simulink model "hems_model"  (R2024b)
settings: Solver=ode3  StartTime=0.0  StopTime=86400  FixedStep=900  RelTol=1e-3
values from neighbouring files (symbols this model uses):
  A_win = 15    [hems_init.m]
  bat_cap = 10000    [hems_init.m]
  bat_eff_1way = sqrt(bat_eff)    [hems_init.m]
  bat_soc0 = 5000    [hems_init.m]
  C_bldg = 8000 * 3600    (= 28800000)    [hems_init.m]
  C_tank = V_tank*rho_w*c_w    (= 1255800)    [hems_init.m]
  dr_power = 2500    [hems_init.m]
  g_val = 0.55    [hems_init.m]
  H_T = 128    [hems_init.m]
  Q_int = 600    [hems_init.m]
  T_in0 = 20    [hems_init.m]
  T_tank0 = 55    [hems_init.m]
  UA_tank = 2.5    [hems_init.m]
  wm_power = 1500    [hems_init.m]
libraries: simulink x2
settings Model: Creator=orakanti1997  LastModifiedBy=orakanti1997

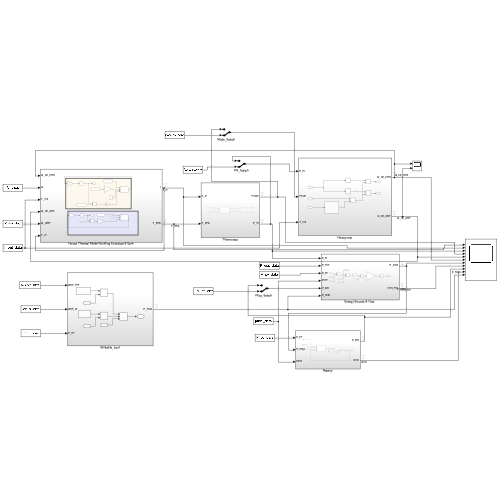
[thumbnail: Simulink's stored preview of the top-level diagram]
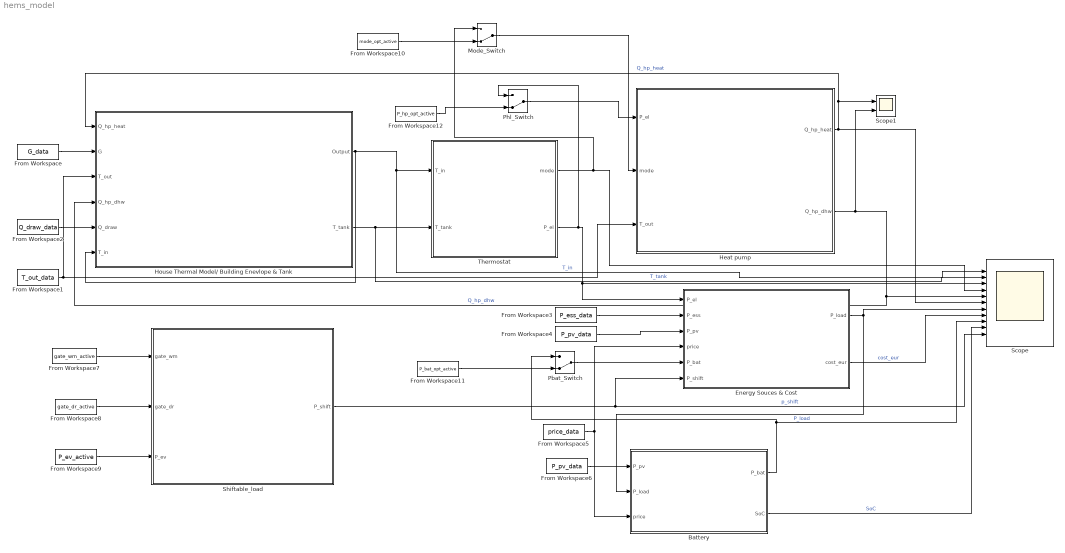
== system hems_model ==
  Battery : Subsystem
  "Energy Souces & Cost " : Subsystem
  From Workspace : FromWorkspace  VariableName=G_data  SampleTime=900
  From Workspace1 : FromWorkspace  VariableName=T_out_data  SampleTime=900
  From Workspace10 : FromWorkspace  VariableName=mode_opt_active
  From Workspace11 : FromWorkspace  VariableName=P_bat_opt_active
  From Workspace12 : FromWorkspace  VariableName=P_hp_opt_active
  From Workspace2 : FromWorkspace  VariableName=Q_draw_data  SampleTime=900
  From Workspace3 : FromWorkspace  VariableName=P_ess_data
  From Workspace4 : FromWorkspace  VariableName=P_pv_data
  From Workspace5 : FromWorkspace  VariableName=price_data
  From Workspace6 : FromWorkspace  VariableName=P_pv_data
  From Workspace7 : FromWorkspace  VariableName=gate_wm_active
  From Workspace8 : FromWorkspace  VariableName=gate_dr_active
  From Workspace9 : FromWorkspace  VariableName=P_ev_active
  Heat pump : Subsystem
  House Thermal Model/ Building Enevlope & Tank : Subsystem
  Mode_Switch : ManualSwitch  CurrentSetting=0
  Pbat_Switch : ManualSwitch  CurrentSetting=0
  Phl_Switch : ManualSwitch  CurrentSetting=0
  Scope : Scope  NumInputPorts=11
  Scope1 : Scope  NumInputPorts=2
  Shiftable_load : Subsystem
  Thermostat : Subsystem
  wires:
  Battery/1(P_bat) -> Pbat_Switch/1, Scope/9
  "Energy Souces & Cost "/2(cost_eur) -> Scope/8  "cost_eur"
  Heat pump/2(Q_hp_dhw) -> House Thermal Model/ Building Enevlope & Tank/4(Q_hp_dhw), Scope/5, Scope1/2  "Q_hp_dhw"
  Shiftable_load/1(P_shift) -> "Energy Souces & Cost "/6(P_shift), Scope/11  "p_shift"
  From Workspace5/1 -> "Energy Souces & Cost "/4(price), Battery/3(price)
  From Workspace4/1 -> "Energy Souces & Cost "/3(P_pv)
  "Energy Souces & Cost "/1(P_load) -> Battery/2(P_load), Scope/7  "P_load"
  Heat pump/1(Q_hp_heat) -> Scope1/1, House Thermal Model/ Building Enevlope & Tank/1(Q_hp_heat), Scope/6  "Q_hp_heat"
  From Workspace/1 -> House Thermal Model/ Building Enevlope & Tank/2(G)
  From Workspace3/1 -> "Energy Souces & Cost "/2(P_ess)
  From Workspace6/1 -> Battery/1(P_pv)
  Thermostat/1(mode) -> Mode_Switch/1, Scope/4
  From Workspace9/1 -> Shiftable_load/3(P_ev)
  From Workspace7/1 -> Shiftable_load/1(gate_wm)
  House Thermal Model/ Building Enevlope & Tank/2(T_tank) -> Thermostat/2(T_tank), Scope/2  "T_tank"
  From Workspace8/1 -> Shiftable_load/2(gate_dr)
  House Thermal Model/ Building Enevlope & Tank/1(Output) -> Thermostat/1(T_in), Scope/1, House Thermal Model/ Building Enevlope & Tank/6(T_in)  "T_in"
  Thermostat/2(P_el) -> Phl_Switch/1, Scope/3, "Energy Souces & Cost "/1(P_el)
  From Workspace1/1 -> Heat pump/3(T_out), House Thermal Model/ Building Enevlope & Tank/3(T_out)
  Battery/2(SoC) -> Scope/10  "SoC"
  From Workspace2/1 -> House Thermal Model/ Building Enevlope & Tank/5(Q_draw)
  Mode_Switch/1 -> Heat pump/2(mode)
  From Workspace10/1 -> Mode_Switch/2
  Pbat_Switch/1 -> "Energy Souces & Cost "/5(P_bat)
  From Workspace11/1 -> Pbat_Switch/2
  Phl_Switch/1 -> Heat pump/1(P_el)
  From Workspace12/1 -> Phl_Switch/2

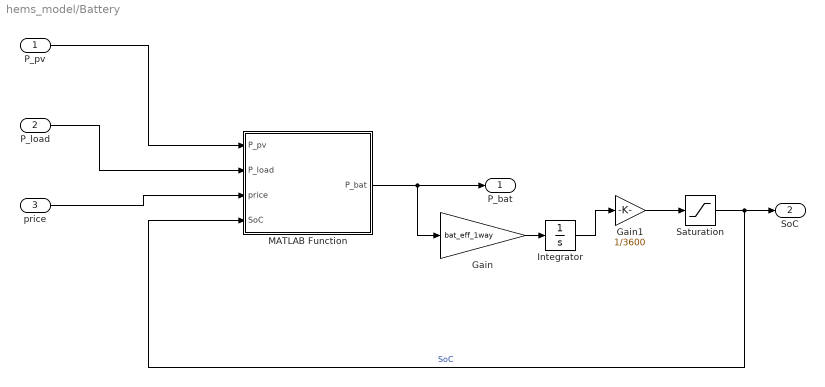
== system hems_model/Battery ==
  P_pv : Inport
  P_load : Inport  Port=2
  price : Inport  Port=3
  Gain : Gain  Gain=bat_eff_1way
  Gain1 : Gain  Gain=1/3600
  Integrator : Integrator  InitialCondition=bat_soc0
  MATLAB Function : MATLAB Function  TreatAsAtomicUnit=on
  Saturation : Saturate  UpperLimit=0.95*bat_cap  LowerLimit=0.10*bat_cap
  P_bat : Outport
  SoC : Outport  Port=2
  wires:
  P_pv/1 -> MATLAB Function/1(P_pv)
  P_load/1 -> MATLAB Function/2(P_load)
  price/1 -> MATLAB Function/3(price)
  Saturation/1 -> MATLAB Function/4(SoC), SoC/1  "SoC"
  MATLAB Function/1(P_bat) -> Gain/1, P_bat/1
  Integrator/1 -> Gain1/1
  Gain1/1 -> Saturation/1
  Gain/1 -> Integrator/1

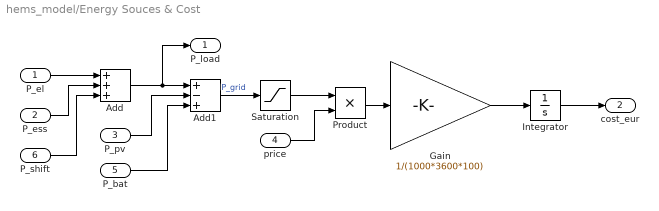
== system hems_model/Energy Souces & Cost  ==
  P_el : Inport
  P_ess : Inport  Port=2
  P_pv : Inport  Port=3
  price : Inport  Port=4
  P_bat : Inport  Port=5
  P_shift : Inport  Port=6
  Add : Sum  Inputs=+++
  Add1 : Sum  Inputs=+-+
  Gain : Gain  Gain=1/(1000*3600*100)
  Integrator : Integrator
  Product : Product
  Saturation : Saturate  UpperLimit=inf  LowerLimit=0
  P_load : Outport
  cost_eur : Outport  Port=2
  wires:
  Product/1 -> Gain/1
  price/1 -> Product/2
  Saturation/1 -> Product/1
  Integrator/1 -> cost_eur/1
  P_pv/1 -> Add1/2
  Gain/1 -> Integrator/1
  P_bat/1 -> Add1/3
  Add/1 -> P_load/1, Add1/1
  P_shift/1 -> Add/3
  P_ess/1 -> Add/2
  Add1/1 -> Saturation/1  "P_grid"
  P_el/1 -> Add/1

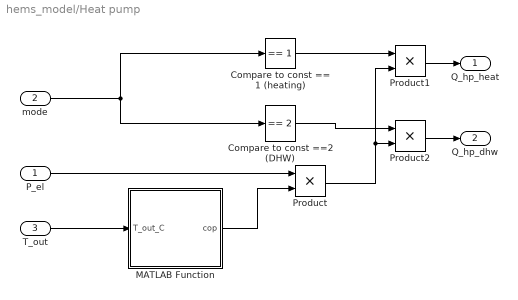
== system hems_model/Heat pump ==
  P_el : Inport
  mode : Inport  Port=2
  T_out : Inport  Port=3
  Compare to const == 1 (heating) : simulink/Logic and Bit Operations/Compare To Constant  relop===  const=1  OutDataTypeStr=uint8
  "Compare to const ==2 (DHW) " : simulink/Logic and Bit Operations/Compare To Constant  relop===  const=2  OutDataTypeStr=uint8
  MATLAB Function : MATLAB Function  TreatAsAtomicUnit=on
  Product : Product
  Product1 : Product
  Product2 : Product
  Q_hp_heat : Outport
  Q_hp_dhw : Outport  Port=2
  wires:
  Product1/1 -> Q_hp_heat/1
  Product/1 -> Product1/2, Product2/2
  Product2/1 -> Q_hp_dhw/1
  MATLAB Function/1(cop) -> Product/2
  Compare to const == 1 (heating)/1 -> Product1/1
  "Compare to const ==2 (DHW) "/1 -> Product2/1
  P_el/1 -> Product/1
  mode/1 -> Compare to const == 1 (heating)/1, "Compare to const ==2 (DHW) "/1
  T_out/1 -> MATLAB Function/1(T_out_C)

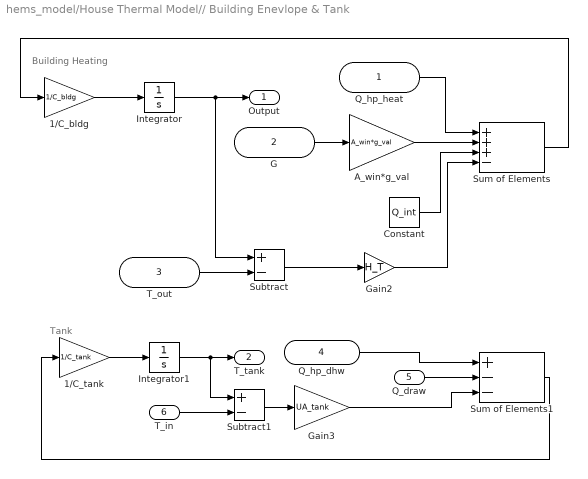
== system hems_model/House Thermal Model// Building Enevlope & Tank ==
  note: Building Heating
  note: Tank
  Q_hp_heat : Inport
  G : Inport  Port=2
  T_out : Inport  Port=3
  Q_hp_dhw : Inport  Port=4
  Q_draw : Inport  Port=5
  T_in : Inport  Port=6
  1/C_bldg : Gain  Gain=1/C_bldg
  1/C_tank : Gain  Gain=1/C_tank
  A_win*g_val : Gain  Gain=A_win*g_val
  Constant : Constant  Value=Q_int
  Gain2 : Gain  Gain=H_T
  Gain3 : Gain  Gain=UA_tank
  Integrator : Integrator  InitialCondition=T_in0
  Integrator1 : Integrator  InitialCondition=T_tank0
  Subtract : Sum  Inputs=+-
  Subtract1 : Sum  Inputs=+-
  Sum of Elements : Sum  Inputs=+++-
  Sum of Elements1 : Sum  Inputs=+--
  Output : Outport
  T_tank : Outport  Port=2
  wires:
  Gain2/1 -> Sum of Elements/4
  A_win*g_val/1 -> Sum of Elements/2
  Q_hp_heat/1 -> Sum of Elements/1
  Subtract/1 -> Gain2/1
  G/1 -> A_win*g_val/1
  Integrator/1 -> Subtract/1, Output/1
  Constant/1 -> Sum of Elements/3
  Sum of Elements1/1 -> 1/C_tank/1
  Q_draw/1 -> Sum of Elements1/2
  Gain3/1 -> Sum of Elements1/3
  Q_hp_dhw/1 -> Sum of Elements1/1
  Sum of Elements/1 -> 1/C_bldg/1
  Subtract1/1 -> Gain3/1
  1/C_bldg/1 -> Integrator/1
  Integrator1/1 -> Subtract1/1, T_tank/1
  T_in/1 -> Subtract1/2
  T_out/1 -> Subtract/2
  1/C_tank/1 -> Integrator1/1

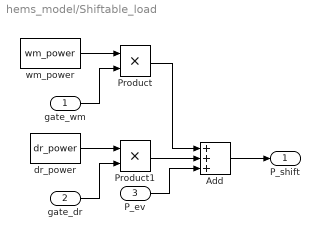
== system hems_model/Shiftable_load ==
  gate_wm : Inport
  gate_dr : Inport  Port=2
  P_ev : Inport  Port=3
  Add : Sum  Inputs=+++
  Product : Product
  Product1 : Product
  dr_power : Constant  Value=dr_power
  wm_power : Constant  Value=wm_power
  P_shift : Outport
  wires:
  P_ev/1 -> Add/3
  Product1/1 -> Add/2
  gate_dr/1 -> Product1/2
  dr_power/1 -> Product1/1
  Add/1 -> P_shift/1
  Product/1 -> Add/1
  gate_wm/1 -> Product/2
  wm_power/1 -> Product/1

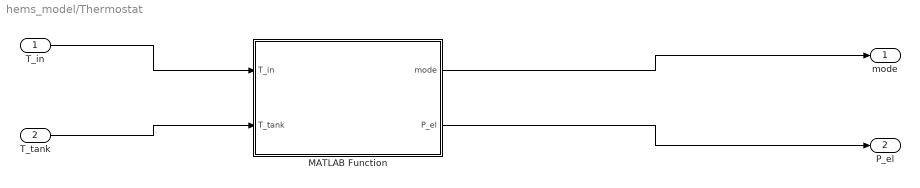
== system hems_model/Thermostat ==
  T_in : Inport
  T_tank : Inport  Port=2
  MATLAB Function : MATLAB Function  TreatAsAtomicUnit=on
  mode : Outport
  P_el : Outport  Port=2
  wires:
  T_in/1 -> MATLAB Function/1(T_in)
  T_tank/1 -> MATLAB Function/2(T_tank)
  MATLAB Function/1(mode) -> mode/1
  MATLAB Function/2(P_el) -> P_el/1

== matlab function hems_model/Thermostat/MATLAB Function ==
  data: T_in input; mode output; T_tank input; P_el output
function [mode, P_el] = thermostat(T_in, T_tank)
    % Rule-based thermostat controller
    % Priority: hot water first, then space heating, else off

    % --- thresholds (hard-coded for now) ---
    T_tank_set = 50;     % tank target [degC]
    T_tank_low = 45;     % tank reheat trigger [degC]
    T_room_set = 21;     % room setpoint [degC]
    T_room_low = 20.5;   % room reheat trigger [degC]
    P_max      = 4000;   % heat pump electrical power [W]

    % --- decision logic ---
    if T_tank < T_tank_low
        mode = 2;            % DHW has priority
    elseif T_in < T_room_low
        mode = 1;            % space heating
    else
        mode = 0;            % off
    end

    % --- power command ---
    if mode == 0
        P_el = 0;
    else
        P_el = P_max;
    end
end

== matlab function hems_model/Heat pump/MATLAB Function ==
  data: T_out_C input; cop output
function cop = calc_cop(T_out_C)
    T_sup_C = 40;          % supply temperature (underfloor heating)
    eta     = 0.45;        % Carnot efficiency factor
    T_out_K = T_out_C + 273.15;
    T_sup_K = T_sup_C + 273.15;
    cop = eta * T_sup_K / (T_sup_K - T_out_K);
    cop = max(min(cop, 6.0), 1.5);   % clamp to physical range
end

== matlab function hems_model/Battery/MATLAB Function ==
  data: P_pv input; P_bat output; P_load input; price input; SoC input
function P_bat = battery_ctrl(P_pv, P_load, price, SoC)
    % Rule-based battery controller
    % P_bat > 0 = charging, P_bat < 0 = discharging

    % --- parameters (hard-coded) ---
    bat_cap     = 10000;   % usable capacity [Wh]
    bat_pmax    = 5000;    % max charge/discharge power [W]
    soc_min     = 0.10 * bat_cap;
    soc_max     = 0.95 * bat_cap;
    price_high  = 28;      % peak-price threshold [ct/kWh]

    surplus = P_pv - P_load;   % >0 means excess solar

    P_bat = 0;   % default: idle

    if surplus > 0 && SoC < soc_max
        % Charge with the solar surplus, capped at max power
        P_bat = min(surplus, bat_pmax);
    elseif price > price_high && SoC > soc_min
        % Discharge during expensive hours to avoid grid import
        P_bat = -bat_pmax;
    end
end
